simulink model "Ivanov_9_airplane"  (Simulink 10.0)
settings: Solver=FixedStepAuto  StartTime=0.0  StopTime=50.0  RelTol=1e-3
undefined symbols (not defined in the file or in its folder): DiscIntNeverNeededParam
libraries: aerolibanim x1
settings Model: Creator=prime  LastModifiedBy=prime
settings DataIOCC: SaveFormat=Dataset  ReturnWorkspaceOutputs=on
settings OptimizationCC: LifeSpan=auto
settings DebuggingCC: UnderspecifiedInitializationDetection=Simplified  MergeDetectMultiDrivingBlocksExec=error  SFUnexpectedBacktrackingDiag=error  SFNoUnconditionalDefaultTransitionDiag=error  SFExecutionAtInitializationDiag=warning  ArithmeticOperatorsInVariantConditions=error
settings HardwareCC: ProdBitPerPointer=64  ProdBitPerSizeT=64  ProdBitPerPtrDiffT=64  ProdLargestAtomicFloat=Float  ProdIntDivRoundTo=Zero  ProdEndianess=LittleEndian  ProdWordSize=64  ProdHWDeviceType=Intel->x86-64 (Windows64)
settings ModelReferenceCC: PropagateSignalLabelsOutOfModel=on
settings SFSimCC: SimUseLocalCustomCode=on  CustomCodeUndefinedFunction=FilterOut
settings RTWCC: RTWUseLocalCustomCode=on
settings CodeAppCC: StateflowObjectComments=off
settings GRTTargetCC: TargetLangStandard=C99 (ISO)  CombineOutputUpdateFcns=on  GRTInterface=off
settings ConfigComp: CovMetricSettings=dwe  CovHtmlReporting=off  CovSaveCumulativeToWorkspaceVar=off  CovSaveSingleToWorkspaceVar=off

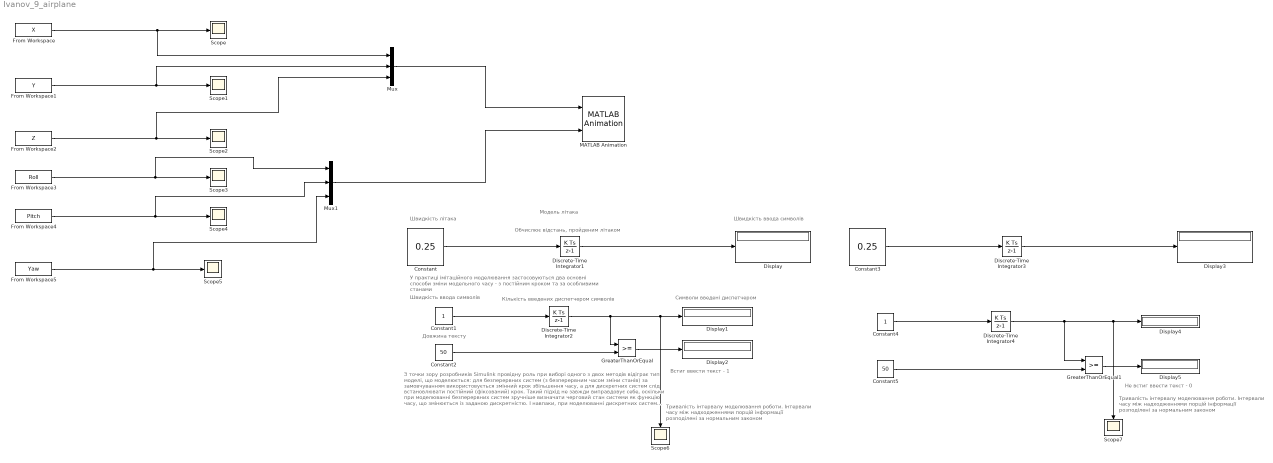
== system Ivanov_9_airplane ==
  note: Символи введені диспетчером
  note: Швидкість ввода символів
  note: Довжина тексту
  note: Швидкість літака
  note: Швидкість ввода символів
  note: Встиг ввести текст - 1
  note: Обчислює відстань, пройденим літаком
  note: Тривалість інтервалу моделювання роботи.
      | Інтервали часу між надходженнями порцій інформації розподілені за нормальним законом
  note: Не встиг ввести текст - 0
  note: Тривалість інтервалу моделювання роботи.
      | Інтервали часу між надходженнями порцій інформації розподілені за нормальним законом
  note: Кількість введених диспетчером символів
  note: У практиці імітаційного моделювання застосовуються два основні способи зміни модельного часу - з постійним кроком та за особливими станами
  note: З точки зору розробників Simulink провідну роль при виборі одного з двох методів відіграє тип моделі, що моделюється: для безперервних систем (з безперервним часом зміни станів) за замовчуванням використовується змінний крок збільшення часу, а для дискретних систем слід встановлювати постійний (фіксований) крок. Такий підхід не завжди виправдовує себе, оскільки при моделюванні безперервних систем зручніше визначати черговий стан системи як функцію часу, що змінюється із заданою дискретністю. І навпаки, при моделюванні дискретних систем величина чергового збільшення часу найчастіше визначається прогнозованим моментом зміни стану системи; причому зміна станів відбувається, зазвичай, нерегулярно. Тому корисно знати, яким чином розробки моделей дискретних систем можна змусити модельний час змінюватися по особливим станам.
  note: Модель літака
  Constant : Constant  Value=0.25  SampleTime=2
  Constant1 : Constant  SampleTime=2
  Constant2 : Constant  Value=50  SampleTime=2
  Constant3 : Constant  Value=0.25  SampleTime=3
  Constant4 : Constant  SampleTime=3
  Constant5 : Constant  Value=50  SampleTime=3
  Discrete-Time Integrator1 : DiscreteIntegrator  SampleTime=2  ICPrevOutput=DiscIntNeverNeededParam  ICPrevScaledInput=DiscIntNeverNeededParam
  Discrete-Time Integrator2 : DiscreteIntegrator  SampleTime=2  ICPrevOutput=DiscIntNeverNeededParam  ICPrevScaledInput=DiscIntNeverNeededParam
  Discrete-Time Integrator3 : DiscreteIntegrator  SampleTime=3  ICPrevOutput=DiscIntNeverNeededParam  ICPrevScaledInput=DiscIntNeverNeededParam
  Discrete-Time Integrator4 : DiscreteIntegrator  SampleTime=3  ICPrevOutput=DiscIntNeverNeededParam  ICPrevScaledInput=DiscIntNeverNeededParam
  Display{,1..5} (6 alike) : Display
      Display settings: Decimation=13
      Display1 settings: Decimation=50
      Display3 settings: Decimation=13
      Display4 settings: Decimation=50
  From Workspace : FromWorkspace  VariableName=X  SampleTime=2
  From Workspace1 : FromWorkspace  VariableName=Y  SampleTime=2
  From Workspace2 : FromWorkspace  VariableName=Z  SampleTime=2
  From Workspace3 : FromWorkspace  VariableName=Roll  SampleTime=2
  From Workspace4 : FromWorkspace  VariableName=Pitch  SampleTime=2
  From Workspace5 : FromWorkspace  VariableName=Yaw  SampleTime=2
  GreaterThanOrEqual : RelationalOperator  OutDataTypeStr=boolean  RndMeth=Simplest
  GreaterThanOrEqual1 : RelationalOperator  OutDataTypeStr=boolean  RndMeth=Simplest
  MATLAB Animation : aerolibanim/MATLAB Animation  Tag=Matlab Animation 6 DOF  Vehicles=1  Geometries='pa24-250_orange.ac'  BoundingBoxCoordinates=[-50,50,-50,50,-50,50]  CameraOffset=[-150,-50,0]  CameraViewAngle=3  SampleTime=0.01  FigurePosition=[1,49,1536,7.664000e+02]
      settings: SourceProductName=Aerospace Blockset  SourceProductBaseCode=AE
  Mux : Mux  Inputs=3
  Mux1 : Mux  Inputs=3
  Scope{,1..7} (8 alike) : Scope
  wires:
  From Workspace5/1 -> Mux1/3, Scope5/1
  From Workspace3/1 -> Mux1/1, Scope3/1
  From Workspace2/1 -> Mux/3, Scope2/1
  Mux1/1 -> MATLAB Animation/2
  From Workspace/1 -> Mux/1, Scope/1
  From Workspace4/1 -> Mux1/2, Scope4/1
  From Workspace1/1 -> Scope1/1, Mux/2
  Mux/1 -> MATLAB Animation/1
  Discrete-Time Integrator1/1 -> Display/1
  Constant/1 -> Discrete-Time Integrator1/1
  Constant1/1 -> Discrete-Time Integrator2/1
  Discrete-Time Integrator2/1 -> GreaterThanOrEqual/1, Scope6/1, Display1/1
  Constant2/1 -> GreaterThanOrEqual/2
  Constant5/1 -> GreaterThanOrEqual1/2
  GreaterThanOrEqual1/1 -> Display5/1
  Discrete-Time Integrator4/1 -> Scope7/1, Display4/1, GreaterThanOrEqual1/1
  Constant4/1 -> Discrete-Time Integrator4/1
  Constant3/1 -> Discrete-Time Integrator3/1
  Discrete-Time Integrator3/1 -> Display3/1
  GreaterThanOrEqual/1 -> Display2/1
